simulink subsystem "PID_SubSystem"  (R2020b)
settings: Solver=VariableStepAuto  StartTime=0.0  StopTime=10.0  RelTol=1e-3
values from neighbouring files (symbols this model uses):
  Kw = 1/Tw    (= 32.6530612245)    [IThLPlantAntiWindup.m]    (also in PIDAntiWindupResonant.m = 5.88235294118)
  Tl = 1/(5*wgc)    (= 0.00108888888889)    [IThLPlantAntiWindup.m]    (also in PIDAntiWindupResonant.m = 1/(10*wgc))
undefined symbols (not defined in the file or in its folder): daq, Kd, Ki, Kp
settings Model: Creator=umberto  LastModifiedBy=umberto

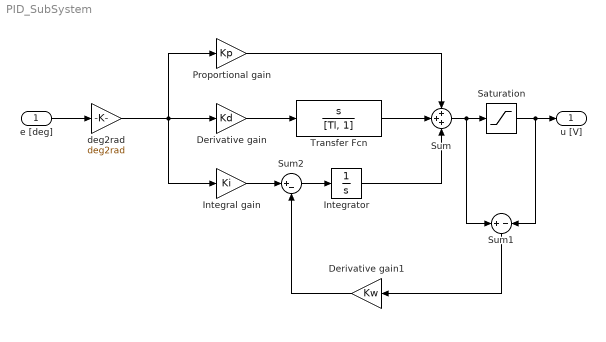
== system PID_SubSystem ==
  e [deg] : Inport
  Derivative gain : Gain  Gain=Kd
  Derivative gain1 : Gain  Gain=Kw
  Integral gain : Gain  Gain=Ki
  Integrator : Integrator
  Proportional gain : Gain  Gain=Kp
  Saturation : Saturate  UpperLimit=daq.dac.fs  LowerLimit=-daq.dac.fs
  Sum : Sum  Inputs=+++
  Sum1 : Sum  Inputs=+|-
  Sum2 : Sum  Inputs=|+-
  Transfer Fcn : TransferFcn  Numerator=[1,0]  Denominator=[Tl, 1]
  deg2rad : Gain  Gain=deg2rad
  u [V] : Outport
  wires:
  Integral gain/1 -> Sum2/1
  Derivative gain/1 -> Transfer Fcn/1
  Integrator/1 -> Sum/3
  Transfer Fcn/1 -> Sum/2
  Proportional gain/1 -> Sum/1
  deg2rad/1 -> Proportional gain/1, Derivative gain/1, Integral gain/1
  e [deg]/1 -> deg2rad/1
  Sum/1 -> Saturation/1, Sum1/1
  Saturation/1 -> u [V]/1, Sum1/2
  Sum1/1 -> Derivative gain1/1
  Derivative gain1/1 -> Sum2/2
  Sum2/1 -> Integrator/1
